simulink model "admittance_control_dyn"  (R2020b)
settings: Solver=FixedStepAuto  StartTime=0.0  StopTime=10  FixedStep=0.001  RelTol=1e-3
undefined symbols (not defined in the file or in its folder): DiscIntNeverNeededParam, Discrete, Time
libraries: simulink x5, ctrlSharedLib x1
settings Model: Creator=fox  LastModifiedBy=fox

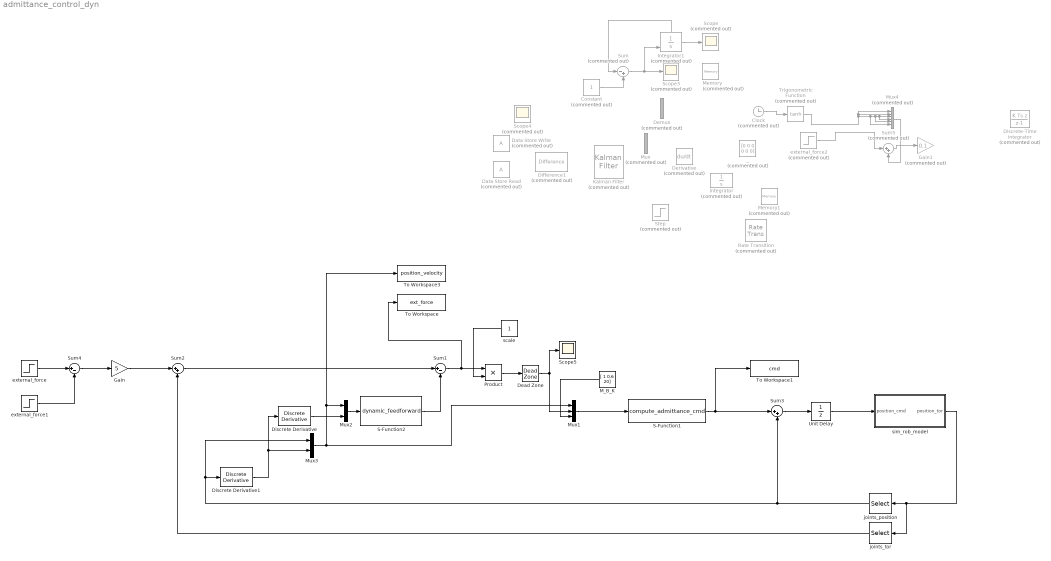
== system admittance_control_dyn ==
  Clock : Clock  Commented=on
  Constant : Constant  Commented=on
  Data Store Read : DataStoreRead  Commented=on
  Data Store Write : DataStoreWrite  Commented=on
  Dead Zone : DeadZone  LowerValue=-2.5  UpperValue=2.5  SaturateOnIntegerOverflow=on
  Demux : Demux  Commented=on  Outputs=2
  Derivative : Derivative  Commented=on
  Difference1 : simulink/Discrete/Difference  Commented=on  ICPrevInput=0.0  OutMin=[]  OutMax=[]  OutDataType=fixdt(1, 16)  OutScaling=2^-10  DoSatur=off
  Discrete Derivative : simulink/Discrete/Discrete Derivative  gainval=1.0  ICPrevScaledInput=0.0  OutMin=[]  OutMax=[]  OutDataType=fixdt(1, 16)  OutScaling=2^-10  DoSatur=off
  Discrete Derivative1 : simulink/Discrete/Discrete Derivative  gainval=1.0  ICPrevScaledInput=0.0  OutMin=[]  OutMax=[]  OutDataType=fixdt(1, 16)  OutScaling=2^-10  DoSatur=off
  Discrete-Time Integrator : DiscreteIntegrator  Commented=on  IntegratorMethod=Integration: Backward Euler  SampleTime=-1  ICPrevOutput=DiscIntNeverNeededParam  ICPrevScaledInput=DiscIntNeverNeededParam
  Gain : Gain  Gain=5
  Gain1 : Gain  Commented=on  Gain=0.1
  Integrator : Integrator  Commented=on
  Integrator1 : Integrator  Commented=on  ExternalReset=falling  ShowStatePort=on
  Kalman Filter : ctrlSharedLib/Kalman Filter  Commented=on  TimeDomain=Discrete-Time  UseCurrentEstimator=on  ModelSource=LTI State-Space Variable  ModelSourceVariable=ss(0.95,1,1,0,1)  A=0.95  B=1  C=1  D=0  NumberOfStates=1  NumberOfInputs=1  NumberOfOutputs=1  InitialEstimateSource=Dialog  X0=0  P0=10  UseK=off  UseGH=off  NumberOfProcessNoiseInputs=1  G=1  TimeInvariantG=on  H=0  TimeInvariantH=on  Q=0.05  TimeInvariantQ=on  R=1  TimeInvariantR=on  N=0  TimeInvariantN=on  AddInputPort=on  AddEnablePort=off  OutputEstimatedY=off  OutputP=off  Ts=-1
  M_B_K : Constant  Value=[ 1 0.6 20]
  Memory : Memory  Commented=on
  Memory1 : Memory  Commented=on  InitialCondition=[0 0 0 0 0 0]
  Mux : Mux  Commented=on  Inputs=2
  Mux1 : Mux  Inputs=3
  Mux2 : Mux  Inputs=2
  Mux3 : Mux  Inputs=2
  Mux4 : Mux  Commented=on  Inputs=6
  Product : Product
  Rate Transition : RateTransition  Commented=on  OutPortSampleTime=1
  S-Function1 : S-Function  FunctionName=compute_admittance_cmd  SFunctionDeploymentMode=off  EnableBusSupport=off
  S-Function2 : S-Function  FunctionName=dynamic_feedforward  SFunctionDeploymentMode=off  EnableBusSupport=off
  Scope : Scope  Commented=on
  Scope3 : Scope  Commented=on
  Scope4 : Scope  Commented=on
  Scope5 : Scope
  Step : Step  Commented=on  SampleTime=0
  Sum : Sum  Commented=on  Inputs=|-+
  Sum1 : Sum  Inputs=|+-
  Sum2 : Sum  Inputs=|++
  Sum3 : Sum  Inputs=|++
  Sum4 : Sum  Inputs=|+-
  Sum5 : Sum  Commented=on  Inputs=|++
  To Workspace : ToWorkspace  VariableName=ext_force  SampleTime=-1
  To Workspace1 : ToWorkspace  VariableName=cmd  SampleTime=-1
  To Workspace3 : ToWorkspace  VariableName=position_velocity  SampleTime=-1
  Trigonometric Function : Trigonometry  Commented=on  Operator=tanh
  Unit Delay : UnitDelay  InitialCondition=[0 0 0 0 0 0]  SampleTime=-1  HasFrameUpgradeWarning=on
  _ : Constant  Commented=on  Value=[0 0 0 0 0 0]
  external_force : Step  Before=[0 0 0 0 0 0]  After="[1  -1 -1 1 1 1]"  SampleTime=0.001
  external_force1 : Step  Time=3  Before=[0 0 0 0 0 0]  After="[1  -1 -1 1 1 1]"  SampleTime=0.001
  external_force2 : Step  Commented=on  Before=[0 0 0 0 0 0]  After=[1 1 1 1 1 1]  SampleTime=0.001
  joints_position : Selector  InputPortWidth=12  IndexOptions=Index vector (dialog)  Indices=[1:6]  OutputSizes=1
  joints_tor : Selector  InputPortWidth=12  IndexOptions=Index vector (dialog)  Indices=[7:12]  OutputSizes=1
  scale : Constant
  sim_rob_model : Subsystem
  wires:
  Integrator1/1 -> Scope/1
  Sum/1 -> Integrator1/2, Scope3/1
  Constant/1 -> Sum/2
  Integrator1/State -> Sum/1
  S-Function2/1 -> Sum1/2
  Sum1/1 -> Product/1, To Workspace/1
  Mux2/1 -> S-Function2/1
  joints_tor/1 -> Sum2/2
  Sum2/1 -> Sum1/1
  M_B_K/1 -> Mux1/3
  Mux3/1 -> Mux1/1, Mux2/1, To Workspace3/1
  Discrete Derivative/1 -> Mux2/2
  Product/1 -> Dead Zone/1
  scale/1 -> Product/2
  Gain/1 -> Sum2/1
  Dead Zone/1 -> Mux1/2, Scope5/1
  Sum4/1 -> Gain/1
  external_force/1 -> Sum4/1
  Mux1/1 -> S-Function1/1
  Trigonometric Function/1 -> Mux4/6, Mux4/5, Mux4/4, Mux4/3, Mux4/2, Mux4/1
  Clock/1 -> Trigonometric Function/1
  Mux4/1 -> Sum5/2
  external_force2/1 -> Sum5/1
  Sum5/1 -> Gain1/1
  sim_rob_model/1(position_tor) -> joints_tor/1, joints_position/1
  joints_position/1 -> Sum3/2, Discrete Derivative1/1, Mux3/1
  Sum3/1 -> Unit Delay/1
  Unit Delay/1 -> sim_rob_model/1(position_cmd)
  S-Function1/1 -> Sum3/1, To Workspace1/1
  Discrete Derivative1/1 -> Mux3/2, Discrete Derivative/1
  external_force1/1 -> Sum4/2

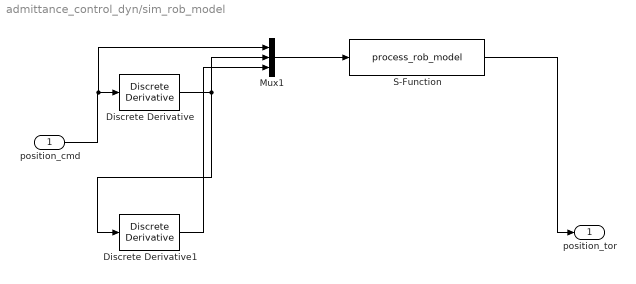
== system admittance_control_dyn/sim_rob_model ==
  position_cmd : Inport
  Discrete Derivative : simulink/Discrete/Discrete Derivative  gainval=1.0  ICPrevScaledInput=0.0  OutMin=[]  OutMax=[]  OutDataType=fixdt(1, 16)  OutScaling=2^-10  DoSatur=off
  Discrete Derivative1 : simulink/Discrete/Discrete Derivative  gainval=1.0  ICPrevScaledInput=0.0  OutMin=[]  OutMax=[]  OutDataType=fixdt(1, 16)  OutScaling=2^-10  DoSatur=off
  Mux1 : Mux  Inputs=3
  S-Function : S-Function  FunctionName=process_rob_model  SFunctionDeploymentMode=off  EnableBusSupport=off
  position_tor : Outport
  wires:
  position_cmd/1 -> Discrete Derivative/1, Mux1/1
  Discrete Derivative/1 -> Discrete Derivative1/1, Mux1/2
  Mux1/1 -> S-Function/1
  S-Function/1 -> position_tor/1
  Discrete Derivative1/1 -> Mux1/3
